simulink model "Simple_4Quad_payload_05"  (R2018b)
settings: Solver=VariableStepAuto  StartTime=0.0  StopTime=60  RelTol=1e-3
InitFcn:
  | Simple_4Quad_payload_05_const
values from neighbouring files (symbols this model uses):
  All_rho = [d1 0 0 ... (first row only)    [Colab_4Quad_model_01_const.m]    (also in Colab_4Quad_model_02_const.m; Simple_4Quad_payload_04_const.m; Simple_4Quad_payload_05_const.m; Simple_4Quad_payload_06_const.m)
  B_ob = [zeros(3);eye(3)]    [Simple_4Quad_payload_04_const.m]    (also in Simple_4Quad_payload_05_const.m; Simple_4Quad_payload_06_const.m; Simple_4Quad_payload_07_const.m; Simple_4Quad_payload_08_const.m)
  BBT_inv = ((B'*B)^(-1))*B'    [Simple_2Quad_payload_03_const.m]    (also in Simple_4Quad_payload_04_const.m = ((BR'*BR)^(-1))*BR'; Simple_4Quad_payload_05_const.m = ((BR'*BR)^(-1))*BR'; Simple_4Quad_payload_06_const.m = ((BR'*BR)^(-1))*BR'; Simple_4Quad_payload_07_const.m = ((BR'*BR)^(-1))*BR')
  BR = 1e0*eye(n)    [Simple_4Quad_payload_04_const.m]    (also in Simple_4Quad_payload_05_const.m; Simple_4Quad_payload_06_const.m; Simple_4Quad_payload_07_const.m; Simple_4Quad_payload_08_const.m)
  C_ob = [eye(3) zeros(3)]    [Simple_4Quad_payload_04_const.m]    (also in Simple_4Quad_payload_05_const.m; Simple_4Quad_payload_06_const.m; Simple_4Quad_payload_07_const.m; Simple_4Quad_payload_08_const.m)
  d1 = 0.25    [Colab_4Quad_model_01_const.m]    (also in Colab_4Quad_model_02_const.m = 0.5; Simple_4Quad_payload_01_const.m = 1; Simple_4Quad_payload_02_const.m = 1; Simple_4Quad_payload_03_const.m = 1)
  d2 = 0.25    [Colab_4Quad_model_01_const.m]    (also in Colab_4Quad_model_02_const.m = 0.5; Simple_4Quad_payload_01_const.m = 1; Simple_4Quad_payload_02_const.m = 1; Simple_4Quad_payload_03_const.m = 1)
  Des_rel_dist = 2    [Simple_4Quad_payload_01_const.m]    (also in Simple_4Quad_payload_02_const.m = 4; Simple_4Quad_payload_03_const.m = 4; Simple_4Quad_payload_04_const.m; Simple_4Quad_payload_05_const.m)
  g = 9.81    [Colab_4Quad_model_01_const.m]    (also in Colab_4Quad_model_02_const.m; Simple_2Quad_payload_01_const.m; Simple_2Quad_payload_02_const.m; Simple_2Quad_payload_03_const.m)
  gamma_0 = 1e-0*diag([1e-3;1e-0])    [Simple_2Quad_payload_03_const.m]    (also in Simple_4Quad_payload_04_const.m = 1e-0*diag([1e-6*ones(3,1);1e-0*ones(3,1)]); Simple_4Quad_payload_05_const.m = 1e-1*diag([1e-6*ones(3,1);1e-0*ones(3,1)]); Simple_4Quad_payload_06_const.m = 1e-0*diag([1e-6*ones(3,1);1e-0*ones(3,1)]); Simple_4Quad_payload_07_const.m = 1e-0*diag([1e-6*ones(3,1);1e-0*ones(3,1)]))
  gamma_1 = 1e+2*diag([1e-3;1e-0])    [Simple_2Quad_payload_03_const.m]    (also in Simple_4Quad_payload_04_const.m = 1e+2*diag([1e-6*ones(3,1);1e-0*ones(3,1)]); Simple_4Quad_payload_05_const.m = 1e+2*diag([1e-6*ones(3,1);1e-0*ones(3,1)]); Simple_4Quad_payload_06_const.m = 1e+3*diag([1e-6*ones(3,1);1e-0*ones(3,1)]); Simple_4Quad_payload_07_const.m = 1e+3*diag([1e-6*ones(3,1);1e-0*ones(3,1)]))
  Ix = 0.166667    [Colab_4Quad_model_01_const.m]    (also in Colab_4Quad_model_02_const.m = 0.02; Simple_4Quad_payload_01_const.m = 1; Simple_4Quad_payload_02_const.m = 1; Simple_4Quad_payload_03_const.m = 1)
  Iy = 0.166667    [Colab_4Quad_model_01_const.m]    (also in Colab_4Quad_model_02_const.m = 0.02; Simple_4Quad_payload_01_const.m = 1; Simple_4Quad_payload_02_const.m = 1; Simple_4Quad_payload_03_const.m = 1)
  Iz = 0.166667    [Colab_4Quad_model_01_const.m]    (also in Colab_4Quad_model_02_const.m = 0.02; Simple_4Quad_payload_01_const.m = 1; Simple_4Quad_payload_02_const.m = 1; Simple_4Quad_payload_03_const.m = 1)
  Jo = diag([Ix;Iy;Iz])    [Colab_4Quad_model_01_const.m]    (also in Colab_4Quad_model_02_const.m; Simple_4Quad_payload_04_const.m; Simple_4Quad_payload_05_const.m; Simple_4Quad_payload_06_const.m)
  Jq = diag([0.0291 0.0291 0.0552])    [Colab_4Quad_model_01_const.m]    (also in Colab_4Quad_model_02_const.m = diag([0.03 0.03 0.06]); Simple_4Quad_payload_03_const.m = 1.2416e-3 * diag([1 1 2]); Simple_4Quad_payload_04_const.m = 1 * diag([1 1 2]); Simple_4Quad_payload_05_const.m = 1 * diag([1 1 2]))
  k1 = 1    [Simple_2Quad_payload_03_const.m]    (also in Simple_4Quad_payload_04_const.m; Simple_4Quad_payload_05_const.m; Simple_4Quad_payload_06_const.m; Simple_4Quad_payload_07_const.m)
  k2 = 0.1    [Simple_2Quad_payload_03_const.m]    (also in Simple_4Quad_payload_04_const.m; Simple_4Quad_payload_05_const.m; Simple_4Quad_payload_06_const.m; Simple_4Quad_payload_07_const.m)
  ki1_N = 0    [Simple_4Quad_payload_02_const.m]    (also in Simple_4Quad_payload_03_const.m; Simple_4Quad_payload_04_const.m; Simple_4Quad_payload_05_const.m; Simple_4Quad_payload_06_const.m)
  ki2_N = 0    [Simple_4Quad_payload_02_const.m]    (also in Simple_4Quad_payload_03_const.m; Simple_4Quad_payload_04_const.m; Simple_4Quad_payload_05_const.m; Simple_4Quad_payload_06_const.m = 10)
  kp1_N = 10    [Simple_4Quad_payload_02_const.m]    (also in Simple_4Quad_payload_03_const.m; Simple_4Quad_payload_04_const.m; Simple_4Quad_payload_05_const.m = 1; Simple_4Quad_payload_06_const.m = 1)
  kp2_N = 100    [Simple_4Quad_payload_02_const.m]    (also in Simple_4Quad_payload_03_const.m; Simple_4Quad_payload_04_const.m; Simple_4Quad_payload_05_const.m = 1; Simple_4Quad_payload_06_const.m = 1)
  l = 3.1819    [Colab_4Quad_model_01_const.m]    (also in Colab_4Quad_model_02_const.m = 3; Simple_2Quad_payload_04_const.m = 1; Simple_4Quad_payload_01_const.m = 1; Simple_4Quad_payload_02_const.m = 2)
  m = 1.5    [Colab_4Quad_model_01_const.m]    (also in Colab_4Quad_model_02_const.m; Simple_2Quad_payload_04_const.m = 1; Simple_4Quad_payload_01_const.m = 1; Simple_4Quad_payload_02_const.m = 1)
  M = 1.0    (= 1)    [Colab_4Quad_model_01_const.m]    (also in Colab_4Quad_model_02_const.m; Simple_2Quad_payload_01_const.m; Simple_2Quad_payload_02_const.m; Simple_2Quad_payload_03_const.m)
  Md = 1*[1;1;1]    [Simple_2Quad_payload_04_const.m]    (also in Simple_4Quad_payload_01_const.m = 1*[1;1;1;1;1;1]; Simple_4Quad_payload_02_const.m = 1*[1;1;1;1;1;1]; Simple_4Quad_payload_03_const.m = 1*[1;1;1;1;1;1]; Simple_4Quad_payload_04_const.m = 1*[1;1;1;1;1;1])
  n = 2    [Simple_2Quad_payload_03_const.m]    (also in Simple_4Quad_payload_03_const.m = 6; Simple_4Quad_payload_04_const.m = 6; Simple_4Quad_payload_05_const.m = 6; Simple_4Quad_payload_06_const.m = 6)
  Q_ob = var_u_ob * eye(6)    [Simple_4Quad_payload_04_const.m]    (also in Simple_4Quad_payload_05_const.m; Simple_4Quad_payload_06_const.m; Simple_4Quad_payload_07_const.m; Simple_4Quad_payload_08_const.m)
  QR = 1e-0*eye(n)    [Simple_4Quad_payload_04_const.m]    (also in Simple_4Quad_payload_05_const.m = 1e-1*eye(n); Simple_4Quad_payload_06_const.m; Simple_4Quad_payload_07_const.m; Simple_4Quad_payload_08_const.m)
  R = 1e+0*eye(n)    [Simple_2Quad_payload_03_const.m]    (also in Simple_4Quad_payload_04_const.m = 1e+0*eye(m); Simple_4Quad_payload_05_const.m = 1e+0*eye(m); Simple_4Quad_payload_06_const.m; Simple_4Quad_payload_07_const.m)
  R_ob = var_y_ob * eye(3)    [Simple_4Quad_payload_04_const.m]    (also in Simple_4Quad_payload_05_const.m; Simple_4Quad_payload_06_const.m; Simple_4Quad_payload_07_const.m; Simple_4Quad_payload_08_const.m)
  rho_0 = 1e-0    (= 1)    [Simple_2Quad_payload_03_const.m]    (also in Simple_4Quad_payload_04_const.m; Simple_4Quad_payload_05_const.m = 0.1; Simple_4Quad_payload_06_const.m; Simple_4Quad_payload_07_const.m)
  rho_1 = 1e-0    (= 1)    [Simple_2Quad_payload_03_const.m]    (also in Simple_4Quad_payload_04_const.m; Simple_4Quad_payload_05_const.m; Simple_4Quad_payload_06_const.m; Simple_4Quad_payload_07_const.m)
libraries: simulink x8
(part 2 of 3)

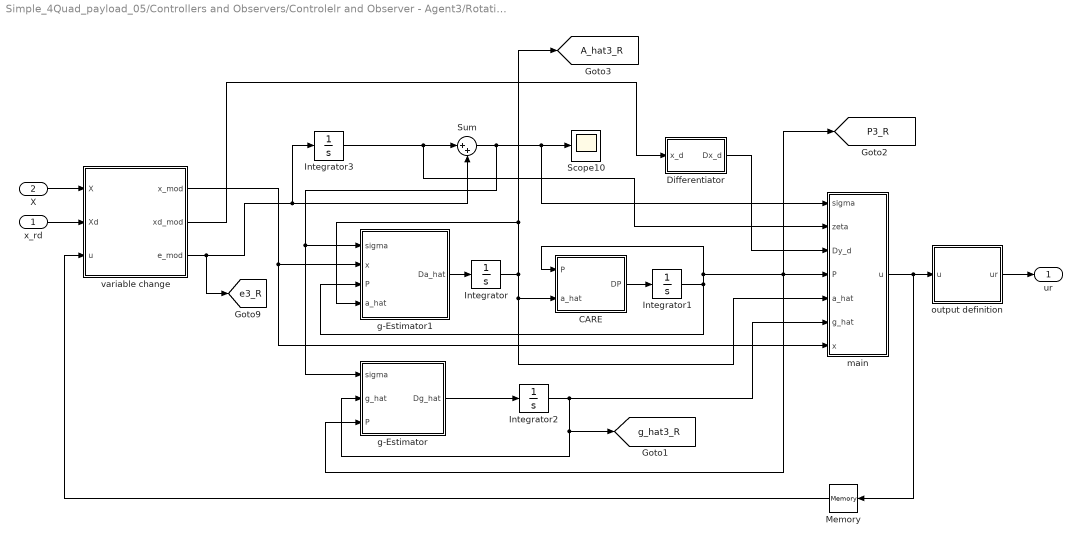
== system Simple_4Quad_payload_05/Controllers and Observers/Controlelr and Observer - Agent3/Rotational #3 ==
  x_rd : Inport
  X : Inport  Port=2
  CARE : MATLAB Function  TreatAsAtomicUnit=on
  Differentiator : Subsystem
  Integrator : Integrator  InitialCondition=zeros(n)
  Integrator1 : Integrator  InitialCondition=eye(n)
  Integrator2 : Integrator  InitialCondition=zeros(n,1)
  Integrator3 : Integrator  InitialCondition=zeros(n,1)
  Memory : Memory  InitialCondition=zeros(n,1)
  Scope10 : Scope
  Sum : Sum  Inputs=|++
  g-Estimator : MATLAB Function  TreatAsAtomicUnit=on
  g-Estimator1 : MATLAB Function  TreatAsAtomicUnit=on
  main : MATLAB Function  TreatAsAtomicUnit=on
  output definition : MATLAB Function  TreatAsAtomicUnit=on
  variable change : MATLAB Function  TreatAsAtomicUnit=on
  ur : Outport
  tag scope: A_hat3_R=global, P3_R=global, e3_R=global, g_hat3_R=global
  wires:
  Integrator2/1 -> g-Estimator/2(g_hat), [g_hat3_R], main/6(g_hat)
  Memory/1 -> variable change/3(u)
  variable change/3(e_mod) -> Integrator3/1, Sum/2, [e3_R]
  variable change/2(xd_mod) -> Differentiator/1(x_d)
  Integrator3/1 -> Sum/1, main/2(zeta)
  main/1(u) -> output definition/1(u), Memory/1
  Differentiator/1(Dx_d) -> main/3(Dy_d)
  g-Estimator/1(Dg_hat) -> Integrator2/1
  Integrator/1 -> main/5(a_hat), CARE/2(a_hat), g-Estimator1/4(a_hat), [A_hat3_R]
  Integrator1/1 -> main/4(P), g-Estimator/3(P), [P3_R], CARE/1(P), g-Estimator1/3(P)
  variable change/1(x_mod) -> g-Estimator1/2(x), main/7(x)
  g-Estimator1/1(Da_hat) -> Integrator/1
  Sum/1 -> g-Estimator1/1(sigma), g-Estimator/1(sigma), Scope10/1, main/1(sigma)
  CARE/1(DP) -> Integrator1/1
  X/1 -> variable change/1(X)
  x_rd/1 -> variable change/2(Xd)
  output definition/1(ur) -> ur/1

== system Simple_4Quad_payload_05/Controllers and Observers/Controller and Observer - Agent2/Observer2 ==
  wo : Inport
  Dwo : Inport  Port=2
  Rel_Pos_local2 : Inport  Port=3
  Rel_Acc_local2 : Inport  Port=4
  Agent_Num : Inport  Port=5
  Integrator : Integrator  InitialCondition=eye(6)
  Integrator1 : Integrator  InitialCondition=[0;0;1;0;0;0]
  Kalman_Filter2 : MATLAB Function  TreatAsAtomicUnit=on
  Observer_Finalization2 : MATLAB Function  TreatAsAtomicUnit=on
  q2_hat : Outport
  Dq2_hat : Outport  Port=2
  tag scope: Dq2_hat=global, q2_hat=global
  wires:
  Kalman_Filter2/1(DP_ob) -> Integrator/1
  Kalman_Filter2/2(Dxhat_ob) -> Integrator1/1
  Integrator/1 -> Kalman_Filter2/1(P_ob)
  Integrator1/1 -> Kalman_Filter2/2(xhat_ob), Observer_Finalization2/1(xhati)
  wo/1 -> Kalman_Filter2/3(wo)
  Dwo/1 -> Kalman_Filter2/4(Dwo)
  Rel_Pos_local2/1 -> Kalman_Filter2/5(Rel_Posi_local)
  Rel_Acc_local2/1 -> Kalman_Filter2/6(Rel_Acci_local)
  Agent_Num/1 -> Kalman_Filter2/7(Agent_Num)
  Observer_Finalization2/1(qhati) -> [q2_hat], q2_hat/1
  Observer_Finalization2/2(Dqhati) -> [Dq2_hat], Dq2_hat/1

== system Simple_4Quad_payload_05/Controllers and Observers/Controller and Observer - Agent2/PID_q2 ==
  q2_des : Inport
  q2 : Inport  Port=2
  Dq2 : Inport  Port=3
  PID Controller : simulink/Continuous/PID Controller  Controller=PID  Form=Parallel  TimeDomain=Continuous-time  SampleTime=-1  IntegratorMethod=Forward Euler  FilterMethod=Forward Euler  ControllerParametersSource=internal  P=kp1_N  I=ki1_N  D=0  UseFilter=on  N=100  TunerSelectOption=Transfer Function Based (PID Tuner App)  InitialConditionSource=internal  InitialConditionForIntegrator=0  InitialConditionForFilter=0  DifferentiatorICPrevScaledInput=0  ExternalReset=none  TrackingMode=off  Kt=1  LimitOutput=off  UpperSaturationLimit=inf  LowerSaturationLimit=-inf  LinearizeAsGain=on  AntiWindupMode=none  Kb=1  POutMin=[]  POutMax=[]  IOutMin=[]  IOutMax=[]  DOutMin=[]  DOutMax=[]  NOutMin=[]  NOutMax=[]  SumOutMin=[]  SumOutMax=[]  SaturationOutMin=[]  SaturationOutMax=[]  PParamMin=[]  PParamMax=[]  IParamMin=[]  IParamMax=[]  DParamMin=[]  DParamMax=[]  NParamMin=[]  NParamMax=[]  KbParamMin=[]  KbParamMax=[]  KtParamMin=[]  KtParamMax=[]  KbOutMin=[]  KbOutMax=[]  KtOutMin=[]  KtOutMax=[]  IntegratorOutMin=[]  IntegratorOutMax=[]  FilterOutMin=[]  FilterOutMax=[]  SumI1OutMin=[]  SumI1OutMax=[]  SumI2OutMin=[]  SumI2OutMax=[]  SumI3OutMin=[]  SumI3OutMax=[]  SumI4OutMin=[]  SumI4OutMax=[]  SumDOutMin=[]  SumDOutMax=[]  DifferentiatorOutMin=[]  DifferentiatorOutMax=[]  FilterDiffOutCoefMin=[]  FilterDiffOutCoefMax=[]  ReciprocalOutMin=[]  ReciprocalOutMax=[]  SumDenOutMin=[]  SumDenOutMax=[]  SumNumOutMin=[]  SumNumOutMax=[]  DivideOutMin=[]  DivideOutMax=[]  IntegratorContinuousStateAttributes=''  IntegratorStateMustResolveToSignalObject=off  IntegratorRTWStateStorageClass=Auto  FilterContinuousStateAttributes=''  FilterStateMustResolveToSignalObject=off  FilterRTWStateStorageClass=Auto  ParallelPVariant=InternalParameters  IdealPVariant=Disabled  IVariant=InternalParameters  DVariant=InternalParameters  IntegratorVariant=Continuous  SatVariant=Disabled  AWVariant=Passthrough  PCopyVariant=Disabled  TRVariant=Disabled  FdbkBlocksVariant=Forward  IdealPFdbkVariant=Disabled  SatFdbkVariant=Disabled  DerivativeFilterVariant=ContFilter  NVariant=InternalParameters  NCopyVariant=Disabled  FilterICVariant=InternalICsFilter  IntegratorICVariant=InternalICs  ExternalResetVariant=Disabled  TRSumVariant=Passthrough  SumFdbkVariant=Disabled  SumVariant=Sum_PID
  PID Controller1 : simulink/Continuous/PID Controller  Controller=PID  Form=Parallel  TimeDomain=Continuous-time  SampleTime=-1  IntegratorMethod=Forward Euler  FilterMethod=Forward Euler  ControllerParametersSource=internal  P=kp2_N  I=ki2_N  D=0  UseFilter=on  N=100  TunerSelectOption=Transfer Function Based (PID Tuner App)  InitialConditionSource=internal  InitialConditionForIntegrator=0  InitialConditionForFilter=0  DifferentiatorICPrevScaledInput=0  ExternalReset=none  TrackingMode=off  Kt=1  LimitOutput=off  UpperSaturationLimit=inf  LowerSaturationLimit=-inf  LinearizeAsGain=on  AntiWindupMode=none  Kb=1  POutMin=[]  POutMax=[]  IOutMin=[]  IOutMax=[]  DOutMin=[]  DOutMax=[]  NOutMin=[]  NOutMax=[]  SumOutMin=[]  SumOutMax=[]  SaturationOutMin=[]  SaturationOutMax=[]  PParamMin=[]  PParamMax=[]  IParamMin=[]  IParamMax=[]  DParamMin=[]  DParamMax=[]  NParamMin=[]  NParamMax=[]  KbParamMin=[]  KbParamMax=[]  KtParamMin=[]  KtParamMax=[]  KbOutMin=[]  KbOutMax=[]  KtOutMin=[]  KtOutMax=[]  IntegratorOutMin=[]  IntegratorOutMax=[]  FilterOutMin=[]  FilterOutMax=[]  SumI1OutMin=[]  SumI1OutMax=[]  SumI2OutMin=[]  SumI2OutMax=[]  SumI3OutMin=[]  SumI3OutMax=[]  SumI4OutMin=[]  SumI4OutMax=[]  SumDOutMin=[]  SumDOutMax=[]  DifferentiatorOutMin=[]  DifferentiatorOutMax=[]  FilterDiffOutCoefMin=[]  FilterDiffOutCoefMax=[]  ReciprocalOutMin=[]  ReciprocalOutMax=[]  SumDenOutMin=[]  SumDenOutMax=[]  SumNumOutMin=[]  SumNumOutMax=[]  DivideOutMin=[]  DivideOutMax=[]  IntegratorContinuousStateAttributes=''  IntegratorStateMustResolveToSignalObject=off  IntegratorRTWStateStorageClass=Auto  FilterContinuousStateAttributes=''  FilterStateMustResolveToSignalObject=off  FilterRTWStateStorageClass=Auto  ParallelPVariant=InternalParameters  IdealPVariant=Disabled  IVariant=InternalParameters  DVariant=InternalParameters  IntegratorVariant=Continuous  SatVariant=Disabled  AWVariant=Passthrough  PCopyVariant=Disabled  TRVariant=Disabled  FdbkBlocksVariant=Forward  IdealPFdbkVariant=Disabled  SatFdbkVariant=Disabled  DerivativeFilterVariant=ContFilter  NVariant=InternalParameters  NCopyVariant=Disabled  FilterICVariant=InternalICsFilter  IntegratorICVariant=InternalICs  ExternalResetVariant=Disabled  TRSumVariant=Passthrough  SumFdbkVariant=Disabled  SumVariant=Sum_PID
  Sum : Sum  Inputs=|+-
  Sum1 : Sum  Inputs=|+-
  N2 : Outport
  wires:
  Dq2/1 -> Sum1/2
  q2/1 -> Sum/2
  q2_des/1 -> Sum/1
  Sum1/1 -> PID Controller1/1
  Sum/1 -> PID Controller/1
  PID Controller1/1 -> N2/1
  PID Controller/1 -> Sum1/1

== system Simple_4Quad_payload_05/Controllers and Observers/Controller and Observer - Agent2/Rotation_Q2 ==
  Omega Q2 : Inport
  D Phi : MATLAB Function  TreatAsAtomicUnit=on
  Integrator : Integrator  InitialCondition=zeros(3,1)
  Mux : Mux  Inputs=2
  X_Rot_Q2 : Outport
  wires:
  D Phi/1(D_PHI_Q2) -> Integrator/1
  Omega Q2/1 -> Mux/2, D Phi/1(Omega_Q2)
  Integrator/1 -> D Phi/2(PHI_Q2), Mux/1
  Mux/1 -> X_Rot_Q2/1

== system Simple_4Quad_payload_05/Controllers and Observers/Controller and Observer - Agent2/Rotational #2 ==
  x_rd : Inport
  X : Inport  Port=2
  CARE : MATLAB Function  TreatAsAtomicUnit=on
  Differentiator : Subsystem
  Integrator : Integrator  InitialCondition=zeros(n)
  Integrator1 : Integrator  InitialCondition=eye(n)
  Integrator2 : Integrator  InitialCondition=zeros(n,1)
  Integrator3 : Integrator  InitialCondition=zeros(n,1)
  Memory : Memory  InitialCondition=zeros(n,1)
  Scope10 : Scope
  Sum : Sum  Inputs=|++
  g-Estimator : MATLAB Function  TreatAsAtomicUnit=on
  g-Estimator1 : MATLAB Function  TreatAsAtomicUnit=on
  main : MATLAB Function  TreatAsAtomicUnit=on
  output definition : MATLAB Function  TreatAsAtomicUnit=on
  variable change : MATLAB Function  TreatAsAtomicUnit=on
  ur : Outport
  tag scope: A_hat2_R=global, P2_R=global, e2_R=global, g_hat2_R=global
  wires:
  x_rd/1 -> variable change/2(Xd)
  X/1 -> variable change/1(X)
  CARE/1(DP) -> Integrator1/1
  Sum/1 -> main/1(sigma), Scope10/1, g-Estimator/1(sigma), g-Estimator1/1(sigma)
  g-Estimator1/1(Da_hat) -> Integrator/1
  variable change/1(x_mod) -> main/7(x), g-Estimator1/2(x)
  Integrator1/1 -> g-Estimator1/3(P), CARE/1(P), [P2_R], g-Estimator/3(P), main/4(P)
  Integrator/1 -> [A_hat2_R], g-Estimator1/4(a_hat), CARE/2(a_hat), main/5(a_hat)
  g-Estimator/1(Dg_hat) -> Integrator2/1
  Differentiator/1(Dx_d) -> main/3(Dy_d)
  main/1(u) -> Memory/1, output definition/1(u)
  Integrator3/1 -> main/2(zeta), Sum/1
  variable change/2(xd_mod) -> Differentiator/1(x_d)
  variable change/3(e_mod) -> [e2_R], Sum/2, Integrator3/1
  Memory/1 -> variable change/3(u)
  Integrator2/1 -> main/6(g_hat), [g_hat2_R], g-Estimator/2(g_hat)
  output definition/1(ur) -> ur/1

== system Simple_4Quad_payload_05/Controllers and Observers/Controller and Observer - Agent4/Observer4 ==
  wo : Inport
  Dwo : Inport  Port=2
  Rel_Pos_local4 : Inport  Port=3
  Rel_Acc_local4 : Inport  Port=4
  Agent_Num : Inport  Port=5
  Integrator : Integrator  InitialCondition=eye(6)
  Integrator1 : Integrator  InitialCondition=[0;0;1;0;0;0]
  Kalman_Filter4 : MATLAB Function  TreatAsAtomicUnit=on
  Observer_Finalization4 : MATLAB Function  TreatAsAtomicUnit=on
  q4_hat : Outport
  Dq4_hat : Outport  Port=2
  tag scope: Dq4_hat=global, q4_hat=global
  wires:
  Kalman_Filter4/1(DP_ob) -> Integrator/1
  Kalman_Filter4/2(Dxhat_ob) -> Integrator1/1
  Integrator/1 -> Kalman_Filter4/1(P_ob)
  Integrator1/1 -> Observer_Finalization4/1(xhati), Kalman_Filter4/2(xhat_ob)
  wo/1 -> Kalman_Filter4/3(wo)
  Dwo/1 -> Kalman_Filter4/4(Dwo)
  Rel_Pos_local4/1 -> Kalman_Filter4/5(Rel_Posi_local)
  Rel_Acc_local4/1 -> Kalman_Filter4/6(Rel_Acci_local)
  Agent_Num/1 -> Kalman_Filter4/7(Agent_Num)
  Observer_Finalization4/1(qhati) -> [q4_hat], q4_hat/1
  Observer_Finalization4/2(Dqhati) -> [Dq4_hat], Dq4_hat/1

== system Simple_4Quad_payload_05/Controllers and Observers/Controller and Observer - Agent4/PID_q4 ==
  q4_des : Inport
  q4 : Inport  Port=2
  Dq4 : Inport  Port=3
  PID Controller : simulink/Continuous/PID Controller  Controller=PID  Form=Parallel  TimeDomain=Continuous-time  SampleTime=-1  IntegratorMethod=Forward Euler  FilterMethod=Forward Euler  ControllerParametersSource=internal  P=kp1_N  I=ki1_N  D=0  UseFilter=on  N=100  TunerSelectOption=Transfer Function Based (PID Tuner App)  InitialConditionSource=internal  InitialConditionForIntegrator=0  InitialConditionForFilter=0  DifferentiatorICPrevScaledInput=0  ExternalReset=none  TrackingMode=off  Kt=1  LimitOutput=off  UpperSaturationLimit=inf  LowerSaturationLimit=-inf  LinearizeAsGain=on  AntiWindupMode=none  Kb=1  POutMin=[]  POutMax=[]  IOutMin=[]  IOutMax=[]  DOutMin=[]  DOutMax=[]  NOutMin=[]  NOutMax=[]  SumOutMin=[]  SumOutMax=[]  SaturationOutMin=[]  SaturationOutMax=[]  PParamMin=[]  PParamMax=[]  IParamMin=[]  IParamMax=[]  DParamMin=[]  DParamMax=[]  NParamMin=[]  NParamMax=[]  KbParamMin=[]  KbParamMax=[]  KtParamMin=[]  KtParamMax=[]  KbOutMin=[]  KbOutMax=[]  KtOutMin=[]  KtOutMax=[]  IntegratorOutMin=[]  IntegratorOutMax=[]  FilterOutMin=[]  FilterOutMax=[]  SumI1OutMin=[]  SumI1OutMax=[]  SumI2OutMin=[]  SumI2OutMax=[]  SumI3OutMin=[]  SumI3OutMax=[]  SumI4OutMin=[]  SumI4OutMax=[]  SumDOutMin=[]  SumDOutMax=[]  DifferentiatorOutMin=[]  DifferentiatorOutMax=[]  FilterDiffOutCoefMin=[]  FilterDiffOutCoefMax=[]  ReciprocalOutMin=[]  ReciprocalOutMax=[]  SumDenOutMin=[]  SumDenOutMax=[]  SumNumOutMin=[]  SumNumOutMax=[]  DivideOutMin=[]  DivideOutMax=[]  IntegratorContinuousStateAttributes=''  IntegratorStateMustResolveToSignalObject=off  IntegratorRTWStateStorageClass=Auto  FilterContinuousStateAttributes=''  FilterStateMustResolveToSignalObject=off  FilterRTWStateStorageClass=Auto  ParallelPVariant=InternalParameters  IdealPVariant=Disabled  IVariant=InternalParameters  DVariant=InternalParameters  IntegratorVariant=Continuous  SatVariant=Disabled  AWVariant=Passthrough  PCopyVariant=Disabled  TRVariant=Disabled  FdbkBlocksVariant=Forward  IdealPFdbkVariant=Disabled  SatFdbkVariant=Disabled  DerivativeFilterVariant=ContFilter  NVariant=InternalParameters  NCopyVariant=Disabled  FilterICVariant=InternalICsFilter  IntegratorICVariant=InternalICs  ExternalResetVariant=Disabled  TRSumVariant=Passthrough  SumFdbkVariant=Disabled  SumVariant=Sum_PID
  PID Controller1 : simulink/Continuous/PID Controller  Controller=PID  Form=Parallel  TimeDomain=Continuous-time  SampleTime=-1  IntegratorMethod=Forward Euler  FilterMethod=Forward Euler  ControllerParametersSource=internal  P=kp2_N  I=ki2_N  D=0  UseFilter=on  N=100  TunerSelectOption=Transfer Function Based (PID Tuner App)  InitialConditionSource=internal  InitialConditionForIntegrator=0  InitialConditionForFilter=0  DifferentiatorICPrevScaledInput=0  ExternalReset=none  TrackingMode=off  Kt=1  LimitOutput=off  UpperSaturationLimit=inf  LowerSaturationLimit=-inf  LinearizeAsGain=on  AntiWindupMode=none  Kb=1  POutMin=[]  POutMax=[]  IOutMin=[]  IOutMax=[]  DOutMin=[]  DOutMax=[]  NOutMin=[]  NOutMax=[]  SumOutMin=[]  SumOutMax=[]  SaturationOutMin=[]  SaturationOutMax=[]  PParamMin=[]  PParamMax=[]  IParamMin=[]  IParamMax=[]  DParamMin=[]  DParamMax=[]  NParamMin=[]  NParamMax=[]  KbParamMin=[]  KbParamMax=[]  KtParamMin=[]  KtParamMax=[]  KbOutMin=[]  KbOutMax=[]  KtOutMin=[]  KtOutMax=[]  IntegratorOutMin=[]  IntegratorOutMax=[]  FilterOutMin=[]  FilterOutMax=[]  SumI1OutMin=[]  SumI1OutMax=[]  SumI2OutMin=[]  SumI2OutMax=[]  SumI3OutMin=[]  SumI3OutMax=[]  SumI4OutMin=[]  SumI4OutMax=[]  SumDOutMin=[]  SumDOutMax=[]  DifferentiatorOutMin=[]  DifferentiatorOutMax=[]  FilterDiffOutCoefMin=[]  FilterDiffOutCoefMax=[]  ReciprocalOutMin=[]  ReciprocalOutMax=[]  SumDenOutMin=[]  SumDenOutMax=[]  SumNumOutMin=[]  SumNumOutMax=[]  DivideOutMin=[]  DivideOutMax=[]  IntegratorContinuousStateAttributes=''  IntegratorStateMustResolveToSignalObject=off  IntegratorRTWStateStorageClass=Auto  FilterContinuousStateAttributes=''  FilterStateMustResolveToSignalObject=off  FilterRTWStateStorageClass=Auto  ParallelPVariant=InternalParameters  IdealPVariant=Disabled  IVariant=InternalParameters  DVariant=InternalParameters  IntegratorVariant=Continuous  SatVariant=Disabled  AWVariant=Passthrough  PCopyVariant=Disabled  TRVariant=Disabled  FdbkBlocksVariant=Forward  IdealPFdbkVariant=Disabled  SatFdbkVariant=Disabled  DerivativeFilterVariant=ContFilter  NVariant=InternalParameters  NCopyVariant=Disabled  FilterICVariant=InternalICsFilter  IntegratorICVariant=InternalICs  ExternalResetVariant=Disabled  TRSumVariant=Passthrough  SumFdbkVariant=Disabled  SumVariant=Sum_PID
  Sum : Sum  Inputs=|+-
  Sum1 : Sum  Inputs=|+-
  N4 : Outport
  wires:
  Dq4/1 -> Sum1/2
  q4/1 -> Sum/2
  q4_des/1 -> Sum/1
  Sum1/1 -> PID Controller1/1
  Sum/1 -> PID Controller/1
  PID Controller1/1 -> N4/1
  PID Controller/1 -> Sum1/1

== system Simple_4Quad_payload_05/Controllers and Observers/Controller and Observer - Agent4/Rotation_Q4 ==
  Omega Q4 : Inport
  D Phi : MATLAB Function  TreatAsAtomicUnit=on
  Integrator : Integrator  InitialCondition=zeros(3,1)
  Mux : Mux  Inputs=2
  X_Rot_Q4 : Outport
  wires:
  D Phi/1(D_PHI_Q4) -> Integrator/1
  Omega Q4/1 -> Mux/2, D Phi/1(Omega_Q4)
  Integrator/1 -> D Phi/2(PHI_Q4), Mux/1
  Mux/1 -> X_Rot_Q4/1

== system Simple_4Quad_payload_05/Controllers and Observers/Controller and Observer - Agent4/Rotational #4 ==
  x_rd : Inport
  X : Inport  Port=2
  CARE : MATLAB Function  TreatAsAtomicUnit=on
  Differentiator : Subsystem
  Integrator : Integrator  InitialCondition=zeros(n)
  Integrator1 : Integrator  InitialCondition=eye(n)
  Integrator2 : Integrator  InitialCondition=zeros(n,1)
  Integrator3 : Integrator  InitialCondition=zeros(n,1)
  Memory : Memory  InitialCondition=zeros(n,1)
  Scope10 : Scope
  Sum : Sum  Inputs=|++
  g-Estimator : MATLAB Function  TreatAsAtomicUnit=on
  g-Estimator1 : MATLAB Function  TreatAsAtomicUnit=on
  main : MATLAB Function  TreatAsAtomicUnit=on
  output definition : MATLAB Function  TreatAsAtomicUnit=on
  variable change : MATLAB Function  TreatAsAtomicUnit=on
  ur : Outport
  tag scope: A_hat4_R=global, P4_R=global, e4_R=global, g_hat4_R=global
  wires:
  x_rd/1 -> variable change/2(Xd)
  X/1 -> variable change/1(X)
  CARE/1(DP) -> Integrator1/1
  Sum/1 -> main/1(sigma), Scope10/1, g-Estimator/1(sigma), g-Estimator1/1(sigma)
  g-Estimator1/1(Da_hat) -> Integrator/1
  variable change/1(x_mod) -> main/7(x), g-Estimator1/2(x)
  Integrator1/1 -> g-Estimator1/3(P), CARE/1(P), [P4_R], g-Estimator/3(P), main/4(P)
  Integrator/1 -> [A_hat4_R], g-Estimator1/4(a_hat), CARE/2(a_hat), main/5(a_hat)
  g-Estimator/1(Dg_hat) -> Integrator2/1
  Differentiator/1(Dx_d) -> main/3(Dy_d)
  main/1(u) -> Memory/1, output definition/1(u)
  Integrator3/1 -> main/2(zeta), Sum/1
  variable change/2(xd_mod) -> Differentiator/1(x_d)
  variable change/3(e_mod) -> [e4_R], Sum/2, Integrator3/1
  Memory/1 -> variable change/3(u)
  Integrator2/1 -> main/6(g_hat), [g_hat4_R], g-Estimator/2(g_hat)
  output definition/1(ur) -> ur/1

== system Simple_4Quad_payload_05/Controllers and Observers/Cotnroller and Observer - Agent1 /Observer1 ==
  wo : Inport
  Dwo : Inport  Port=2
  Rel_Pos_local1 : Inport  Port=3
  Rel_Acc_local1 : Inport  Port=4
  Agent_Num : Inport  Port=5
  Integrator : Integrator  InitialCondition=eye(6)
  Integrator1 : Integrator  InitialCondition=[0;0;1;0;0;0]
  Kalman_Filter1 : MATLAB Function  TreatAsAtomicUnit=on
  Observer_Finalization1 : MATLAB Function  TreatAsAtomicUnit=on
  q1_hat : Outport
  Dq1_hat : Outport  Port=2
  tag scope: Dq1_hat=global, q1_hat=global
  wires:
  Kalman_Filter1/1(DP_ob) -> Integrator/1
  Kalman_Filter1/2(Dxhat_ob) -> Integrator1/1
  Integrator/1 -> Kalman_Filter1/1(P_ob)
  Integrator1/1 -> Kalman_Filter1/2(xhat_ob), Observer_Finalization1/1(xhati)
  wo/1 -> Kalman_Filter1/3(wo)
  Dwo/1 -> Kalman_Filter1/4(Dwo)
  Observer_Finalization1/1(qhati) -> [q1_hat], q1_hat/1
  Observer_Finalization1/2(Dqhati) -> [Dq1_hat], Dq1_hat/1
  Rel_Pos_local1/1 -> Kalman_Filter1/5(Rel_Posi_local)
  Rel_Acc_local1/1 -> Kalman_Filter1/6(Rel_Acci_local)
  Agent_Num/1 -> Kalman_Filter1/7(Agent_Num)

== system Simple_4Quad_payload_05/Controllers and Observers/Cotnroller and Observer - Agent1 /PID_q1 ==
  q1_des : Inport
  q1 : Inport  Port=2
  Dq1 : Inport  Port=3
  PID Controller : simulink/Continuous/PID Controller  Controller=PID  Form=Parallel  TimeDomain=Continuous-time  SampleTime=-1  IntegratorMethod=Forward Euler  FilterMethod=Forward Euler  ControllerParametersSource=internal  P=kp1_N  I=ki1_N  D=0  UseFilter=on  N=100  TunerSelectOption=Transfer Function Based (PID Tuner App)  InitialConditionSource=internal  InitialConditionForIntegrator=0  InitialConditionForFilter=0  DifferentiatorICPrevScaledInput=0  ExternalReset=none  TrackingMode=off  Kt=1  LimitOutput=off  UpperSaturationLimit=inf  LowerSaturationLimit=-inf  LinearizeAsGain=on  AntiWindupMode=none  Kb=1  POutMin=[]  POutMax=[]  IOutMin=[]  IOutMax=[]  DOutMin=[]  DOutMax=[]  NOutMin=[]  NOutMax=[]  SumOutMin=[]  SumOutMax=[]  SaturationOutMin=[]  SaturationOutMax=[]  PParamMin=[]  PParamMax=[]  IParamMin=[]  IParamMax=[]  DParamMin=[]  DParamMax=[]  NParamMin=[]  NParamMax=[]  KbParamMin=[]  KbParamMax=[]  KtParamMin=[]  KtParamMax=[]  KbOutMin=[]  KbOutMax=[]  KtOutMin=[]  KtOutMax=[]  IntegratorOutMin=[]  IntegratorOutMax=[]  FilterOutMin=[]  FilterOutMax=[]  SumI1OutMin=[]  SumI1OutMax=[]  SumI2OutMin=[]  SumI2OutMax=[]  SumI3OutMin=[]  SumI3OutMax=[]  SumI4OutMin=[]  SumI4OutMax=[]  SumDOutMin=[]  SumDOutMax=[]  DifferentiatorOutMin=[]  DifferentiatorOutMax=[]  FilterDiffOutCoefMin=[]  FilterDiffOutCoefMax=[]  ReciprocalOutMin=[]  ReciprocalOutMax=[]  SumDenOutMin=[]  SumDenOutMax=[]  SumNumOutMin=[]  SumNumOutMax=[]  DivideOutMin=[]  DivideOutMax=[]  IntegratorContinuousStateAttributes=''  IntegratorStateMustResolveToSignalObject=off  IntegratorRTWStateStorageClass=Auto  FilterContinuousStateAttributes=''  FilterStateMustResolveToSignalObject=off  FilterRTWStateStorageClass=Auto  ParallelPVariant=InternalParameters  IdealPVariant=Disabled  IVariant=InternalParameters  DVariant=InternalParameters  IntegratorVariant=Continuous  SatVariant=Disabled  AWVariant=Passthrough  PCopyVariant=Disabled  TRVariant=Disabled  FdbkBlocksVariant=Forward  IdealPFdbkVariant=Disabled  SatFdbkVariant=Disabled  DerivativeFilterVariant=ContFilter  NVariant=InternalParameters  NCopyVariant=Disabled  FilterICVariant=InternalICsFilter  IntegratorICVariant=InternalICs  ExternalResetVariant=Disabled  TRSumVariant=Passthrough  SumFdbkVariant=Disabled  SumVariant=Sum_PID
  PID Controller1 : simulink/Continuous/PID Controller  Controller=PID  Form=Parallel  TimeDomain=Continuous-time  SampleTime=-1  IntegratorMethod=Forward Euler  FilterMethod=Forward Euler  ControllerParametersSource=internal  P=kp2_N  I=ki2_N  D=0  UseFilter=on  N=100  TunerSelectOption=Transfer Function Based (PID Tuner App)  InitialConditionSource=internal  InitialConditionForIntegrator=0  InitialConditionForFilter=0  DifferentiatorICPrevScaledInput=0  ExternalReset=none  TrackingMode=off  Kt=1  LimitOutput=off  UpperSaturationLimit=inf  LowerSaturationLimit=-inf  LinearizeAsGain=on  AntiWindupMode=none  Kb=1  POutMin=[]  POutMax=[]  IOutMin=[]  IOutMax=[]  DOutMin=[]  DOutMax=[]  NOutMin=[]  NOutMax=[]  SumOutMin=[]  SumOutMax=[]  SaturationOutMin=[]  SaturationOutMax=[]  PParamMin=[]  PParamMax=[]  IParamMin=[]  IParamMax=[]  DParamMin=[]  DParamMax=[]  NParamMin=[]  NParamMax=[]  KbParamMin=[]  KbParamMax=[]  KtParamMin=[]  KtParamMax=[]  KbOutMin=[]  KbOutMax=[]  KtOutMin=[]  KtOutMax=[]  IntegratorOutMin=[]  IntegratorOutMax=[]  FilterOutMin=[]  FilterOutMax=[]  SumI1OutMin=[]  SumI1OutMax=[]  SumI2OutMin=[]  SumI2OutMax=[]  SumI3OutMin=[]  SumI3OutMax=[]  SumI4OutMin=[]  SumI4OutMax=[]  SumDOutMin=[]  SumDOutMax=[]  DifferentiatorOutMin=[]  DifferentiatorOutMax=[]  FilterDiffOutCoefMin=[]  FilterDiffOutCoefMax=[]  ReciprocalOutMin=[]  ReciprocalOutMax=[]  SumDenOutMin=[]  SumDenOutMax=[]  SumNumOutMin=[]  SumNumOutMax=[]  DivideOutMin=[]  DivideOutMax=[]  IntegratorContinuousStateAttributes=''  IntegratorStateMustResolveToSignalObject=off  IntegratorRTWStateStorageClass=Auto  FilterContinuousStateAttributes=''  FilterStateMustResolveToSignalObject=off  FilterRTWStateStorageClass=Auto  ParallelPVariant=InternalParameters  IdealPVariant=Disabled  IVariant=InternalParameters  DVariant=InternalParameters  IntegratorVariant=Continuous  SatVariant=Disabled  AWVariant=Passthrough  PCopyVariant=Disabled  TRVariant=Disabled  FdbkBlocksVariant=Forward  IdealPFdbkVariant=Disabled  SatFdbkVariant=Disabled  DerivativeFilterVariant=ContFilter  NVariant=InternalParameters  NCopyVariant=Disabled  FilterICVariant=InternalICsFilter  IntegratorICVariant=InternalICs  ExternalResetVariant=Disabled  TRSumVariant=Passthrough  SumFdbkVariant=Disabled  SumVariant=Sum_PID
  Sum : Sum  Inputs=|+-
  Sum1 : Sum  Inputs=|+-
  N1 : Outport
  wires:
  Dq1/1 -> Sum1/2
  q1/1 -> Sum/2
  q1_des/1 -> Sum/1
  Sum1/1 -> PID Controller1/1
  Sum/1 -> PID Controller/1
  PID Controller1/1 -> N1/1
  PID Controller/1 -> Sum1/1

== system Simple_4Quad_payload_05/Controllers and Observers/Cotnroller and Observer - Agent1 /Rotation_Q1 ==
  Omega Q1 : Inport
  D Phi : MATLAB Function  TreatAsAtomicUnit=on
  Integrator : Integrator  InitialCondition=zeros(3,1)
  Mux : Mux  Inputs=2
  X_Rot_Q1 : Outport
  wires:
  D Phi/1(D_PHI_Q1) -> Integrator/1
  Omega Q1/1 -> D Phi/1(Omega_Q1), Mux/2
  Integrator/1 -> D Phi/2(PHI_Q1), Mux/1
  Mux/1 -> X_Rot_Q1/1

== system Simple_4Quad_payload_05/Controllers and Observers/Cotnroller and Observer - Agent1 /Rotational #1 ==
  x_rd : Inport
  X : Inport  Port=2
  CARE : MATLAB Function  TreatAsAtomicUnit=on
  Differentiator : Subsystem
  Integrator : Integrator  InitialCondition=zeros(n)
  Integrator1 : Integrator  InitialCondition=eye(n)
  Integrator2 : Integrator  InitialCondition=zeros(n,1)
  Integrator3 : Integrator  InitialCondition=zeros(n,1)
  Memory : Memory  InitialCondition=zeros(n,1)
  Sum : Sum  Inputs=|++
  g-Estimator : MATLAB Function  TreatAsAtomicUnit=on
  g-Estimator1 : MATLAB Function  TreatAsAtomicUnit=on
  main : MATLAB Function  TreatAsAtomicUnit=on
  output definition : MATLAB Function  TreatAsAtomicUnit=on
  variable change : MATLAB Function  TreatAsAtomicUnit=on
  ur1 : Outport
  tag scope: A_hat1_R=global, P1_R=global, e1_R=global, g_hat1_R=global
  wires:
  x_rd/1 -> variable change/2(Xd)
  X/1 -> variable change/1(X)
  CARE/1(DP) -> Integrator1/1
  Sum/1 -> main/1(sigma), g-Estimator/1(sigma), g-Estimator1/1(sigma)
  g-Estimator1/1(Da_hat) -> Integrator/1
  variable change/1(x_mod) -> main/7(x), g-Estimator1/2(x)
  Integrator1/1 -> g-Estimator1/3(P), CARE/1(P), [P1_R], g-Estimator/3(P), main/4(P)
  Integrator/1 -> [A_hat1_R], g-Estimator1/4(a_hat), CARE/2(a_hat), main/5(a_hat)
  g-Estimator/1(Dg_hat) -> Integrator2/1
  Differentiator/1(Dx_d) -> main/3(Dy_d)
  main/1(u) -> output definition/1(u), Memory/1
  Integrator3/1 -> main/2(zeta), Sum/1
  variable change/2(xd_mod) -> Differentiator/1(x_d)
  variable change/3(e_mod) -> [e1_R], Sum/2, Integrator3/1
  Memory/1 -> variable change/3(u)
  Integrator2/1 -> main/6(g_hat), [g_hat1_R], g-Estimator/2(g_hat)
  output definition/1(ur) -> ur1/1

== system Simple_4Quad_payload_05/Controllers and Observers/Controlelr and Observer - Agent3/Rotational #3/Differentiator ==
  x_d : Inport
  Integrator : Integrator  InitialCondition=zeros(n,1)
  Integrator1 : Integrator  InitialCondition=zeros(n,1)
  Scope : Scope
  Scope1 : Scope
  Sliding differentiator : MATLAB Function  TreatAsAtomicUnit=on
  Sliding differentiator1 : MATLAB Function  TreatAsAtomicUnit=on
  Sum : Sum  Inputs=|-+
  Dx_d : Outport
  wires:
  Integrator1/1 -> Sum/2
  Sum/1 -> Sliding differentiator1/1(e), Sliding differentiator/2(e), Scope1/1
  x_d/1 -> Sum/1
  Integrator/1 -> Sliding differentiator/1(u1)
  Sliding differentiator1/1(Du1) -> Integrator/1
  Sliding differentiator/1(u) -> Dx_d/1, Integrator1/1, Scope/1

== system Simple_4Quad_payload_05/Controllers and Observers/Controller and Observer - Agent2/Rotational #2/Differentiator ==
  x_d : Inport
  Integrator : Integrator  InitialCondition=zeros(n,1)
  Integrator1 : Integrator  InitialCondition=zeros(n,1)
  Scope : Scope
  Scope1 : Scope
  Sliding differentiator : MATLAB Function  TreatAsAtomicUnit=on
  Sliding differentiator1 : MATLAB Function  TreatAsAtomicUnit=on
  Sum : Sum  Inputs=|-+
  Dx_d : Outport
  wires:
  Sliding differentiator/1(u) -> Scope/1, Integrator1/1, Dx_d/1
  Sliding differentiator1/1(Du1) -> Integrator/1
  Integrator/1 -> Sliding differentiator/1(u1)
  x_d/1 -> Sum/1
  Sum/1 -> Scope1/1, Sliding differentiator/2(e), Sliding differentiator1/1(e)
  Integrator1/1 -> Sum/2

== system Simple_4Quad_payload_05/Controllers and Observers/Controller and Observer - Agent4/Rotational #4/Differentiator ==
  x_d : Inport
  Integrator : Integrator  InitialCondition=zeros(n,1)
  Integrator1 : Integrator  InitialCondition=zeros(n,1)
  Scope : Scope
  Scope1 : Scope
  Sliding differentiator : MATLAB Function  TreatAsAtomicUnit=on
  Sliding differentiator1 : MATLAB Function  TreatAsAtomicUnit=on
  Sum : Sum  Inputs=|-+
  Dx_d : Outport
  wires:
  Sliding differentiator/1(u) -> Scope/1, Integrator1/1, Dx_d/1
  Sliding differentiator1/1(Du1) -> Integrator/1
  Integrator/1 -> Sliding differentiator/1(u1)
  x_d/1 -> Sum/1
  Sum/1 -> Scope1/1, Sliding differentiator/2(e), Sliding differentiator1/1(e)
  Integrator1/1 -> Sum/2

== system Simple_4Quad_payload_05/Controllers and Observers/Cotnroller and Observer - Agent1 /Rotational #1/Differentiator ==
  x_d : Inport
  Integrator : Integrator  InitialCondition=zeros(n,1)
  Integrator1 : Integrator  InitialCondition=zeros(n,1)
  Sliding differentiator : MATLAB Function  TreatAsAtomicUnit=on
  Sliding differentiator1 : MATLAB Function  TreatAsAtomicUnit=on
  Sum : Sum  Inputs=|-+
  Dx_d : Outport
  wires:
  Sliding differentiator/1(u) -> Integrator1/1, Dx_d/1
  Sliding differentiator1/1(Du1) -> Integrator/1
  Integrator/1 -> Sliding differentiator/1(u1)
  x_d/1 -> Sum/1
  Sum/1 -> Sliding differentiator/2(e), Sliding differentiator1/1(e)
  Integrator1/1 -> Sum/2

== matlab function Simple_4Quad_payload_05/Controllers and Observers/Controller - Payload/Controller ==
  data: e input; F_des output; q_des output; PHI input; Md parameter; g parameter; M parameter; OUT output; d1 parameter; d2 parameter; Ix parameter; Iy parameter; Iz parameter; l parameter; Des_rel_dist parameter
function [F_des,q_des,OUT] = fcn(e,PHI, Md, g, M, d1, d2, Ix, Iy, Iz, l, Des_rel_dist)

phi = PHI(1);
theta = PHI(2);
psi = PHI(3);

Io = diag([Ix;Iy;Iz]);

Ro = [cos(psi)*cos(theta) cos(psi)*sin(theta)*sin(phi)-sin(psi)*cos(phi) cos(psi)*sin(theta)*cos(phi)+sin(psi)*sin(phi);
    sin(psi)*cos(theta) sin(psi)*sin(theta)*sin(phi)+cos(psi)*cos(phi) sin(psi)*sin(theta)*cos(phi)-cos(psi)*sin(phi);
    -sin(theta) cos(theta)*sin(phi) cos(theta)*cos(phi)];

s1 = [0 0 0;
    0 0 -d1;
    0 d1 0];

s2 = [0 0 0;
    0 0 d1;
    0 -d1 0];

s3 = [0 0 d2;
    0 0 0;
    -d2 0 0];

s4 = [0 0 -d2;
    0 0 0;
    d2 0 0];

B = [(1/M)*Ro (1/M)*Ro (1/M)*Ro (1/M)*Ro;
    Io^(-1)*s1 Io^(-1)*s2 Io^(-1)*s3 Io^(-1)*s4;
    1 0 0 1 0 0 0 0 0 0 0 0;
    0 0 0 0 0 0 0 1 0 0 1 0;
    1 0 0 0 0 0 0 0 0 0 0 0;
    0 0 0 0 0 0 0 1 0 0 0 0];

D = [0;0;-g;0;0;0];

SGN = zeros(6);
for i=1:6
    SGN(i,i) = e(i)/(abs(e(i))+0.1);
end

Z = SGN*Md;
U = Z - D;

u_t = U(1:3);
rx_des = Des_rel_dist;
ry_des = Des_rel_dist;
q1 = (rx_des - (2*d1)) / (2*l);
q2 = (ry_des - (2*d2)) / (2*l);
K1 = sqrt( ((u_t(2)/2)^2 + (u_t(3)/4)^2) / ((1/(q1^2))-1) );
K2 = sqrt( ((u_t(1)/2)^2 + (u_t(3)/4)^2) / ((1/(q2^2))-1) );

U_gen = [U;0;0;K1;K2];

Mu = B' * (B*B')^(-1) * U_gen;

F_des = zeros(4,1);
q_des = zeros(3,4);

for i=1:4
    F_des(i,1) = sqrt( Mu((3*(i-1)+1):(3*(i-1)+3))'*Mu((3*(i-1)+1):(3*(i-1)+3)) );
    q_des(:,i) = Mu((3*(i-1)+1):(3*(i-1)+3)) / F_des(i,1);
end

OUT = U;

end

== matlab function Simple_4Quad_payload_05/Controllers and Observers/Cotnroller and Observer - Agent1 /Rotation_Q1/D Phi ==
  data: Omega_Q1 input; D_PHI_Q1 output; PHI_Q1 input
function D_PHI_Q1 = fcn(Omega_Q1,PHI_Q1)

phi_q1 = PHI_Q1(1);
theta_q1 = PHI_Q1(2);

Rm_Q1 = [1 0 -sin(theta_q1);
    0 cos(phi_q1) cos(theta_q1)*sin(phi_q1);
    0 -sin(phi_q1) cos(theta_q1)*cos(phi_q1)];

D_PHI_Q1 = (Rm_Q1)^(-1) * Omega_Q1;


end

== matlab function Simple_4Quad_payload_05/Controllers and Observers/Controller and Observer - Agent2/Dynamic Model2 ==
  data: N2 input; f2 input; q2 input; Dq2 input; m parameter; g parameter; DD_PHI input; DD_P input; D_PHI input; l parameter; PHI input; Agent_Num input; U2_local output; U2 output; All_rho parameter
function [U2_local,U2]  = fcn(N2,f2,q2,Dq2,m, g,DD_PHI,DD_P,D_PHI, l,PHI,Agent_Num,All_rho)

phi = PHI(1);
theta = PHI(2);
psi = PHI(3);

Dist_locali = All_rho(Agent_Num,:)';

Ro = [cos(psi)*cos(theta) cos(psi)*sin(theta)*sin(phi)-sin(psi)*cos(phi) cos(psi)*sin(theta)*cos(phi)+sin(psi)*sin(phi);
    sin(psi)*cos(theta) sin(psi)*sin(theta)*sin(phi)+cos(psi)*cos(phi) sin(psi)*sin(theta)*cos(phi)-cos(psi)*sin(phi);
    -sin(theta) cos(theta)*sin(phi) cos(theta)*cos(phi)];

C1 = External_Product3(D_PHI,Dist_locali);
C2 = External_Product3(D_PHI,C1);
C3 = External_Product3(DD_PHI,Dist_locali);

C4 = External_Product3(Dq2,Dist_locali);
C5 = External_Product3(Dq2,C4);

a_part = ( ( Ro'*DD_P + C2 + C3 ) ) + C5;

G_local = Ro' * [0;0;-g];

T2 = m*a_part(1) + f2 - m*G_local(1);
U2_local = T2*q2 + N2; %[f2+m*g;0;0;];
U2 = Ro * U2_local;

end

== matlab function Simple_4Quad_payload_05/Controllers and Observers/Cotnroller and Observer - Agent1 /Dynamic Model1 ==
  data: N1 input; f1 input; q1 input; Dq1 input; m parameter; g parameter; DD_PHI input; DD_P input; D_PHI input; l parameter; PHI input; U1_local output; U1 output; Agent_Num input; All_rho parameter
function [U1_local,U1]  = fcn(N1,f1,q1,Dq1,m, g,DD_PHI,DD_P,D_PHI, l,PHI,Agent_Num,All_rho)

phi = PHI(1);
theta = PHI(2);
psi = PHI(3);

Dist_locali = All_rho(Agent_Num,:)';

Ro = [cos(psi)*cos(theta) cos(psi)*sin(theta)*sin(phi)-sin(psi)*cos(phi) cos(psi)*sin(theta)*cos(phi)+sin(psi)*sin(phi);
    sin(psi)*cos(theta) sin(psi)*sin(theta)*sin(phi)+cos(psi)*cos(phi) sin(psi)*sin(theta)*cos(phi)-cos(psi)*sin(phi);
    -sin(theta) cos(theta)*sin(phi) cos(theta)*cos(phi)];

C1 = External_Product3(D_PHI,Dist_locali);
C2 = External_Product3(D_PHI,C1);
C3 = External_Product3(DD_PHI,Dist_locali);

C4 = External_Product3(Dq1,Dist_locali);
C5 = External_Product3(Dq1,C4);

a_part = ( ( Ro'*DD_P + C2 + C3 ) ) + C5;

G_local = Ro' * [0;0;-g];

T1 = m*a_part(1) + f1 - m*G_local(1);
U1_local = T1*q1 + N1; %[f1+m*g;0;0;];
U1 = Ro * U1_local;

end

== matlab function Simple_4Quad_payload_05/Controllers and Observers/Controller and Observer - Agent4/Dynamic Model4 ==
  data: N4 input; f4 input; q4 input; Dq4 input; m parameter; g parameter; DD_PHI input; DD_P input; D_PHI input; l parameter; PHI input; Agent_Num input; U4_local output; U4 output; All_rho parameter
function [U4_local,U4]  = fcn(N4,f4,q4,Dq4,m, g,DD_PHI,DD_P,D_PHI, l, PHI,Agent_Num,All_rho)

phi = PHI(1);
theta = PHI(2);
psi = PHI(3);

Dist_locali = All_rho(Agent_Num,:)';

Ro = [cos(psi)*cos(theta) cos(psi)*sin(theta)*sin(phi)-sin(psi)*cos(phi) cos(psi)*sin(theta)*cos(phi)+sin(psi)*sin(phi);
    sin(psi)*cos(theta) sin(psi)*sin(theta)*sin(phi)+cos(psi)*cos(phi) sin(psi)*sin(theta)*cos(phi)-cos(psi)*sin(phi);
    -sin(theta) cos(theta)*sin(phi) cos(theta)*cos(phi)];

C1 = External_Product3(D_PHI,Dist_locali);
C2 = External_Product3(D_PHI,C1);
C3 = External_Product3(DD_PHI,Dist_locali);

C4 = External_Product3(Dq4,Dist_locali);
C5 = External_Product3(Dq4,C4);

a_part = ( ( Ro'*DD_P + C2 + C3 ) ) + C5;

G_local = Ro' * [0;0;-g];

T4 = m*a_part(1) + f4 - m*G_local(1);
U4_local = T4*q4 + N4; %[f4+m*g;0;0;];
U4 = Ro * U4_local;

end

== matlab function Simple_4Quad_payload_05/Controllers and Observers/Controlelr and Observer - Agent3/Dynamic Model3 ==
  data: N3 input; f3 input; q3 input; Dq3 input; m parameter; g parameter; DD_PHI input; DD_P input; D_PHI input; l parameter; PHI input; Agent_Num input; U3_local output; U3 output; All_rho parameter
function [U3_local,U3]  = fcn(N3,f3,q3,Dq3,m, g,DD_PHI,DD_P,D_PHI, l, PHI,Agent_Num,All_rho)

phi = PHI(1);
theta = PHI(2);
psi = PHI(3);

Dist_locali = All_rho(Agent_Num,:)';

Ro = [cos(psi)*cos(theta) cos(psi)*sin(theta)*sin(phi)-sin(psi)*cos(phi) cos(psi)*sin(theta)*cos(phi)+sin(psi)*sin(phi);
    sin(psi)*cos(theta) sin(psi)*sin(theta)*sin(phi)+cos(psi)*cos(phi) sin(psi)*sin(theta)*cos(phi)-cos(psi)*sin(phi);
    -sin(theta) cos(theta)*sin(phi) cos(theta)*cos(phi)];

C1 = External_Product3(D_PHI,Dist_locali);
C2 = External_Product3(D_PHI,C1);
C3 = External_Product3(DD_PHI,Dist_locali);

C4 = External_Product3(Dq3,Dist_locali);
C5 = External_Product3(Dq3,C4);

a_part = ( ( Ro'*DD_P + C2 + C3 ) ) + C5;

G_local = Ro' * [0;0;-g];

T3 = m*a_part(1) + f3 - m*G_local(1);
U3_local = T3*q3 + N3; %[f3+m*g;0;0;];
U3 = Ro * U3_local;

end

== matlab function Simple_4Quad_payload_05/Relative Positions scopes/MATLAB Function ==
  data: P1 input; e_cons_1 output; P2 input; P3 input; P4 input; e_cons_2 output; e_cons_3 output; e_cons_4 output; Des_rel_dist parameter
function [e_cons_1,e_cons_2,e_cons_3,e_cons_4] = fcn(P1,P2,P3,P4,Des_rel_dist)

Pos_local_1 = [Des_rel_dist/2;0;0];
Pos_local_2 = [-Des_rel_dist/2;0;0];
Pos_local_3 = [0;Des_rel_dist/2;0];
Pos_local_4 = [0;-Des_rel_dist/2;0];

Pos_All = [P1 P2 P3 P4];
Pos_local_All = [Pos_local_1 Pos_local_2 Pos_local_3 Pos_local_4];
e_cons_All = zeros(3,4);

for i=1:4
    for j=1:4
        e_cons_All(:,i) = e_cons_All(:,i) + ( (Pos_All(:,i)-Pos_All(:,j)) - (Pos_local_All(:,i)-Pos_local_All(:,j)) );
    end
end

e_cons_1 = e_cons_All(:,1);
e_cons_2 = e_cons_All(:,2);
e_cons_3 = e_cons_All(:,3);
e_cons_4 = e_cons_All(:,4);

end

== matlab function Simple_4Quad_payload_05/Controllers and Observers/Controller - Payload/MATLAB Function ==
  data: t input; Vd output
function Vd = fcn(t)

fv = 0.2;
rv = 1;
Vdz = 0.2;
Vd = [rv*fv*sin(fv*t);
    -rv*fv*cos(fv*t);
    Vdz];

end
